simulink model "IP4"  (R2025b)
settings: Solver=VariableStepAuto  StartTime=0.0  StopTime=10  RelTol=1e-3
PostLoadFcn:
  | IP4_init
values from neighbouring files (symbols this model uses):
  A = [0, 0, 1, 0 ... (first row only)    [IP2_init.m]    (also in IP3_init.m; IP4_init.m; IP_init.m; pid_demo_init.m = [0, 0, 0)
  B = [0;0;4/ (4 * M + m); 6 / (l * (4 * M + m))]    [IP2_init.m]    (also in IP3_init.m; IP4_init.m; IP_init.m; pid_demo_init.m = [1; kd / (Tf + Ts); ki * Ts])
  C = [1, 0, 0, 0]    [IP2_init.m]    (also in IP3_init.m; IP4_init.m; IP_init.m; pid_demo_init.m = [-kd / (Tf + Ts), Tf / (Tf + Ts), 1])
  D = 0    [IP2_init.m]    (also in IP3_init.m; IP4_init.m; IP_init.m; pid_demo_init.m = 333.833333333)
  init_pos = [0, 0]    [IP2_init.m]    (also in IP3_init.m; IP4_init.m; IP_init.m; robot_velocity_input_init.m = deg2rad([0, -130, -100, -40, 90, 0]))
  K = place(A, B, p)    [IP2_init.m]    (also in IP3_init.m; IP4_init.m; IP_init.m; motor_init.m = 0.09)
  kf = -1 / (C*((A - B*K) \ B))    [IP2_init.m]    (also in IP3_init.m; IP4_init.m; IP_init.m)
  Q = 1e-2    (= 0.01)    [IP3_init.m]    (also in IP4_init.m)
  R = 1e-4    (= 0.0001)    [IP3_init.m]    (also in IP4_init.m; motor_init.m = 0.5; task_controller.m = T(1:3, 1:3))
  robot = get_robot_chain(rigid_body, 'rod','base_link')    [IP2_init.m]    (also in IP3_init.m; IP4_init.m; IP_init.m; rcm_generator.m = block.DialogPrm(1).Data)
  Ts = 1e-2    (= 0.01)    [IP4_init.m]    (also in pid_demo_init.m; rcm_generator.m = block.DialogPrm(2).Data)
undefined symbols (not defined in the file or in its folder): Discrete, Time
libraries: ctrlSharedLib x1, aerolibanimutils x1
settings Model: Creator=Junch  LastModifiedBy=Junch

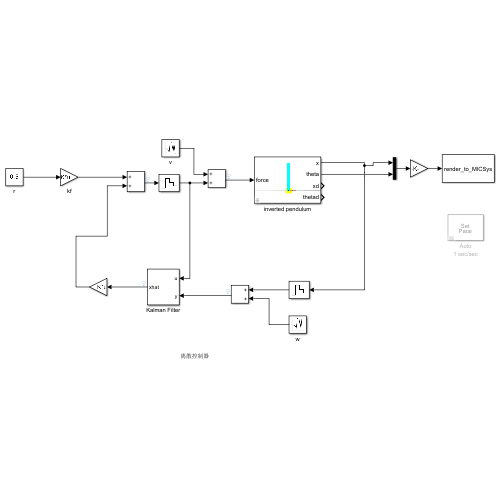
[thumbnail: Simulink's stored preview of the top-level diagram]
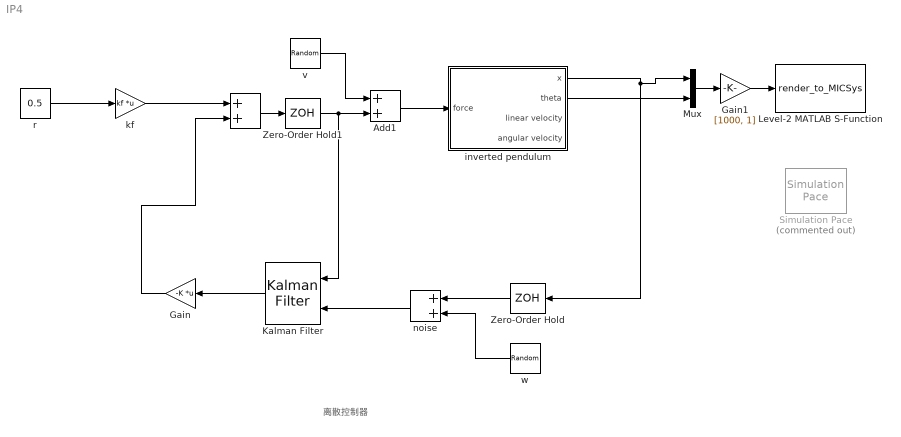
== system IP4 ==
  note: 离散控制器
  " " : Sum
  Add1 : Sum
  Gain : Gain  Gain=-K  Multiplication=Matrix(K*u)
  Gain1 : Gain  Gain=[1000, 1]
  Kalman Filter : ctrlSharedLib/Kalman Filter  TimeDomain=Discrete-Time  UseCurrentEstimator=on  ModelSource=LTI State-Space Variable  ModelSourceVariable=d_plant  A=A  B=B  C=C  D=D  NumberOfStates=1  NumberOfInputs=1  NumberOfOutputs=1  InitialEstimateSource=Dialog  X0=0  P0=10  UseK=off  UseGH=on  NumberOfProcessNoiseInputs=1  G=d_plant.B  TimeInvariantG=on  H=d_plant.D  TimeInvariantH=on  Q=Q  TimeInvariantQ=on  R=R  TimeInvariantR=on  N=0  TimeInvariantN=on  AddInputPort=on  AddEnablePort=off  OutputEstimatedY=off  OutputP=off  Ts=1e-4
  Level-2 MATLAB S-Function : M-S-Function  FunctionName=render_to_MICSys
  Mux : Mux  Inputs=2
  Simulation Pace : aerolibanimutils/Simulation Pace  Commented=on  SimulationPace=1  SleepMode=Auto  OutputPaceError=off  SampleTime=1/30
  Zero-Order Hold : ZeroOrderHold  SampleTime=Ts
  Zero-Order Hold1 : ZeroOrderHold  SampleTime=Ts
  inverted pendulum : Subsystem  mask{robot=robot, init_pos=init_pos, Kd=[0, 0]}
      mask prompts: init_pos "intial position"; Kd "Kd (damping)"
      mask DialogControl ParameterGroupVar Prompt: 参数
      mask Display:
      | image('IP.png');
      | port_label('output', 1, 'x');
      | port_label('output', 2, 'theta');
      | port_label('output', 3, 'xd');
      | port_label('output', 4, 'thetad');
      | port_label('input', 1, 'force');
  kf : Gain  Gain=kf  Multiplication=Matrix(K*u)
  noise : Sum
  r : Constant  Value=0.5  SampleTime=-1
  v : RandomNumber  Variance=Q  SampleTime=Ts
  w : RandomNumber  Variance=R  SampleTime=Ts
  wires:
  Gain1/1 -> Level-2 MATLAB S-Function/1
  inverted pendulum/2(theta) -> Mux/2
  Mux/1 -> Gain1/1
  kf/1 -> " "/1
  r/1 -> kf/1
  inverted pendulum/1(x) -> Zero-Order Hold/1, Mux/1
  Gain/1 -> " "/2
  Add1/1 -> inverted pendulum/1(force)
  " "/1 -> Zero-Order Hold1/1
  v/1 -> Add1/1
  w/1 -> noise/2
  Kalman Filter/1 -> Gain/1
  Zero-Order Hold1/1 -> Kalman Filter/1, Add1/2
  Zero-Order Hold/1 -> noise/1
  noise/1 -> Kalman Filter/2

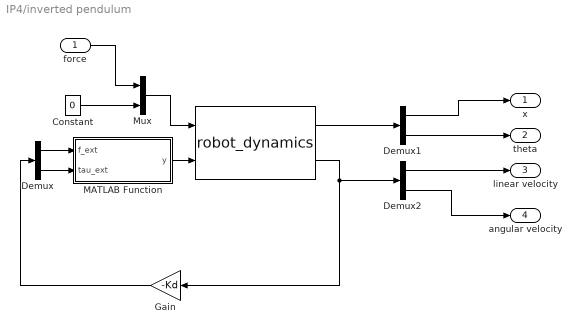
== system IP4/inverted pendulum ==
  force : Inport
  " " : M-S-Function  FunctionName=robot_dynamics  Parameters=robot, init_pos, init_vel  mask{robot=robot, init_pos=init_pos, init_vel=zeros(1,2)}
      mask prompts: robot "robot struct:"; init_pos "init pos:"; init_vel "init velocity:"
      mask DialogControl ParameterGroupVar Prompt: 参数
      mask Display:
      | port_label('input', 1, 'control torque')
      | port_label('input', 2, 'external force')
      | port_label('output', 1, 'q')
      | port_label('output', 2, 'qd')
      | disp('Robot Dynamics');
  Constant : Constant  Value=0
  Demux : Demux  Outputs=2
  Demux1 : Demux  Outputs=2
  Demux2 : Demux  Outputs=2
  Gain : Gain  Gain=-Kd
  MATLAB Function : MATLAB Function  TreatAsAtomicUnit=on
  Mux : Mux  Inputs=2
  x : Outport
  theta : Outport  Port=2
  linear velocity : Outport  Port=3
  angular velocity : Outport  Port=4
  wires:
  Demux/1 -> MATLAB Function/1(f_ext)
  Constant/1 -> Mux/2
  force/1 -> Mux/1
  Gain/1 -> Demux/1
  Mux/1 -> " "/1
  MATLAB Function/1(y) -> " "/2
  " "/2 -> Demux2/1, Gain/1
  Demux/2 -> MATLAB Function/2(tau_ext)
  " "/1 -> Demux1/1
  Demux1/1 -> x/1
  Demux1/2 -> theta/1
  Demux2/1 -> linear velocity/1
  Demux2/2 -> angular velocity/1

== matlab function IP4/inverted pendulum/MATLAB Function ==
  data: f_ext input; y output; tau_ext input
function y = fcn(f_ext, tau_ext)
%#codegen
y1 = [0, 0, 0, f_ext, 0, 0]';
y2 = [0, 0, tau_ext, 0, 0, 0]';
y = [y1, y2];
